simulink model "SL_Practica_4"  (R2024a)
settings: Solver=VariableStepAuto  StartTime=0.0  StopTime=20  RelTol=1e-3
values from neighbouring files (symbols this model uses):
  k = 100    [Parametros_SL_P4.m]    (also in Practica_4.m)
  m = 10    [Parametros_SL_P4.m]    (also in Practica_4.m)
  r = 0.05    [Parametros_SL_P4.m]    (also in Practica_4.m)

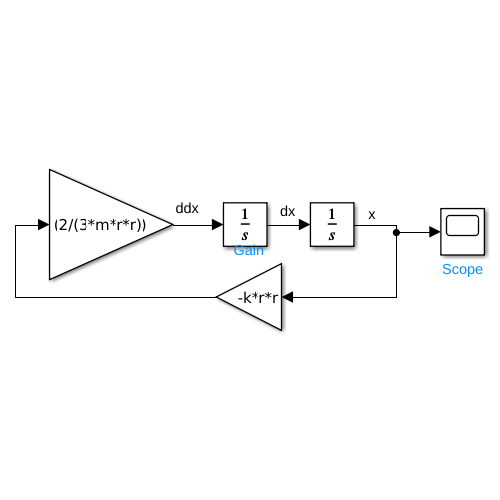
[thumbnail: Simulink's stored preview of the top-level diagram]
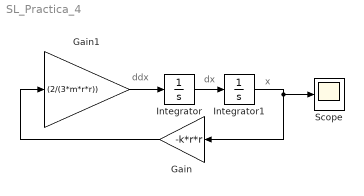
== system SL_Practica_4 ==
  note: x
  note: dx
  note: ddx
  Gain : Gain  Gain=-k*r*r
  Gain1 : Gain  Gain=(2/(3*m*r*r))
  Integrator : Integrator  InitialCondition=2
  Integrator1 : Integrator
  Scope : Scope
  wires:
  Integrator/1 -> Integrator1/1
  Gain1/1 -> Integrator/1
  Integrator1/1 -> Scope/1, Gain/1
  Gain/1 -> Gain1/1
